simulink model "SCR_DAC"  (Simulink 7.9)
settings: Solver=ode45  StartTime=0.0  StopTime=simu.trantime  RelTol=1e-3
undefined symbols (not defined in the file): alpha, beta, Fs, TAO
libraries: simulink x1
settings Model: Creator=amyles  LastModifiedBy=Arnaldi Isacco
settings SolverCC: ZeroCrossAlgorithm=Adaptive  AutoInsertRateTranBlk=on
settings DataIOCC: MaxDataPoints=50000  SaveOutput=off  SaveTime=off
settings OptimizationCC: InlineParams=on
settings DebuggingCC: UnderspecifiedInitializationDetection=Simplified  InvalidFcnCallConnMsg=none  StrictBusMsg=ErrorOnBusTreatedAsVector
settings ModelReferenceCC: ModelReferenceNumInstancesAllowed=Single
settings CodeAppCC: CustomSymbolStrType=$N$R$M_T
settings GRTTargetCC: CombineOutputUpdateFcns=off  GRTInterface=on

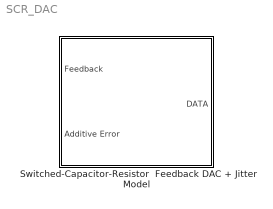
== system SCR_DAC ==
  Switched-Capacitor-Resistor  Feedback DAC + Jitter Model : Subsystem

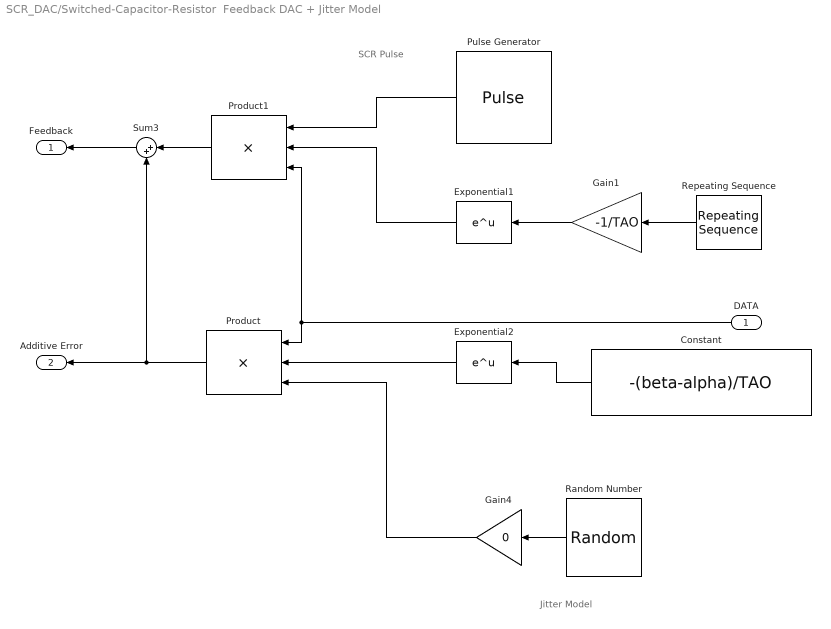
== system SCR_DAC/Switched-Capacitor-Resistor  Feedback DAC + Jitter Model ==
  note: Jitter Model
  note: SCR Pulse
  DATA : Inport
  Constant : Constant  Value=-(beta-alpha)/TAO
  Exponential1 : Math  SampleTime=1/Fs  SaturateOnIntegerOverflow=on
  Exponential2 : Math  SampleTime=1/Fs  SaturateOnIntegerOverflow=on
  Gain1 : Gain  Gain=-1/TAO  SampleTime=1/Fs
  Gain4 : Gain  Gain=0  SampleTime=1/Fs
  Product : Product  Inputs=3  SampleTime=1/Fs  RndMeth=Zero
  Product1 : Product  Inputs=3  SampleTime=1/Fs  RndMeth=Zero
  Pulse Generator : DiscretePulseGenerator  PulseType=Time based  Amplitude=0.5  Period=1/Fs  PulseWidth=25  PhaseDelay=50  SampleTime=1/Fs
  Random Number : RandomNumber  Mean=100e-12  Variance=50e-9  Seed=1  SampleTime=1/Fs
  Repeating Sequence : simulink/Sources/Repeating Sequence  rep_seq_t=[0 1]  rep_seq_y=[0 1]
  Sum3 : Sum  Inputs=|++  SampleTime=1/Fs
  Feedback : Outport
  Additive Error : Outport  Port=2
  wires:
  Pulse Generator/1 -> Product1/1
  Random Number/1 -> Gain4/1
  Product1/1 -> Sum3/1
  Sum3/1 -> Feedback/1
  Gain1/1 -> Exponential1/1
  Exponential1/1 -> Product1/2
  Repeating Sequence/1 -> Gain1/1
  DATA/1 -> Product1/3, Product/1
  Gain4/1 -> Product/3
  Exponential2/1 -> Product/2
  Product/1 -> Sum3/2, Additive Error/1
  Constant/1 -> Exponential2/1
